simulink model "exercise3"  (R2020b)
settings: Solver=VariableStepAuto  StartTime=0.0  StopTime=5  RelTol=1e-3
undefined symbols (not defined in the file): tau
libraries: vrlib x2, dspvision x1
settings Model: OrderedModelArguments=off  Creator=jasper  LastModifiedBy=jasper

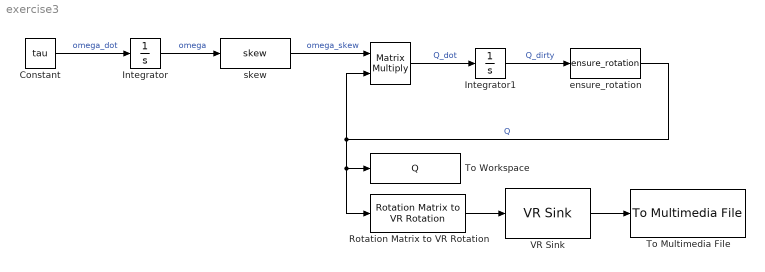
== system exercise3 ==
  " " : Product  Multiplication=Matrix(*)
  Constant : Constant  Value=tau  VectorParams1D=off
  Integrator : Integrator
  Integrator1 : Integrator  InitialCondition=eye(3)
  Rotation Matrix to VR Rotation : vrlib/Utilities/Rotation Matrix to VR Rotation  maxzero=1e-12
      settings: SourceProductBaseCode=SL
  To Multimedia File : dspvision/To Multimedia File  outputFilename=output.avi  streamSelection=Video only  videoCompressor=None (uncompressed)  audioCompressor=None (uncompressed)  imagePorts=One multidimensional signal  fileType=AVI  audioDatatype=Determine from input data type  fourcc=RGB  videoQuality=75  mj2000CompFactor=10
  To Workspace : ToWorkspace  VariableName=Q  SaveFormat=Timeseries  SampleTime=-1
  VR Sink : vrlib/VR Sink  InstantiateOnLoad=on  SampleTime=0.1  ViewEnable=on  RemoteChange=off  RemoteView=off  FieldsWritten=Box.rotation.4.1.1.double  WorldFileName=SingleBox.wrl  AutoView=off  VideoDimensions=[1080 1920]  AllowVariableSize=off  FigureProperties="{'Position', 'Name', 'Viewpoint', 'CameraBound', 'CameraDirection', 'CameraPosition', 'CameraUpVector', 'ZoomFactor', 'Antialiasing', 'Headlight', 'Lighting', 'NavPanel', 'Sound', 'StatusBar', 'Stereo3D', 'Stereo3DCameraOffset', 'Stereo3DHIT', 'ToolBar', 'Textures', 'Transparency', 'Triad', 'Wireframe', 'NavZones', 'NavMode', 'NavSpeed', 'CaptureFileFormat', 'CaptureFileName', 'Record2DCompressMethod', 'Record2DCompressQuality', 'Record2D', 'Record2DFileName', 'Record2DFPS'; [6.9500000000000000e+02   1.1100000000000000e+02   6.4300000000000000e+02   5.7800000000000000e+02], '', 'Camera 1', 'on', [0.0000000000000000e+00   0.0000000000000000e+00  -1.0000000000000000e+00], [0.0000000000000000e+00   0.0000000000000000e+00   0.0000000000000000e+00], [0.0000000000000000e+00   1.0000000000000000e+00   0.0000000000000000e+00], [1.0000000000000000e+00], 'off', 'on', 'on', 'halfbar', 'on', 'on', 'off', [1.0000000149011612e-01], [0.0000000000000000e+00], 'on', 'on', 'on', 'none', 'off', 'off', 'fly', 'normal', 'tif', '%f_anim_%n.tif', 'auto', [7.5000000000000000e+01], 'off', '%f_anim_%n.avi', 'auto'}"
  ensure_rotation : MATLABFcn  MATLABFcn=ensure_rotation  Output1D=off
  skew : MATLABFcn  MATLABFcn=skew  Output1D=off
  wires:
  Constant/1 -> Integrator/1  "omega_dot"
  Integrator/1 -> skew/1  "omega"
  skew/1 -> " "/1  "omega_skew"
  " "/1 -> Integrator1/1  "Q_dot"
  Integrator1/1 -> ensure_rotation/1  "Q_dirty"
  ensure_rotation/1 -> To Workspace/1, Rotation Matrix to VR Rotation/1, " "/2  "Q"
  VR Sink/1 -> To Multimedia File/1
  Rotation Matrix to VR Rotation/1 -> VR Sink/1
